simulink model "sim_sim"  (R2018b)
settings: Solver=ode23s  StartTime=0.0  StopTime=T_sweep  RelTol=1e-3
values from neighbouring files (symbols this model uses):
  dgr = 15    [main_sim.m]    (also in main_sim_exp.m = 0.05; main_sim_exp_2.m = 1.5; main_sim_exp_3.m = 0.65; main_sim_exp_4.m = 12)
  dgs = 1    [main_sim.m]    (also in main_sim_exp.m = 3.5; main_sim_exp_2.m = 3.5; main_sim_exp_3.m = 5; main_sim_exp_4.m = 4.25)
  f_log = 1000    [main_sim.m]    (also in main_sim_exp.m; main_sim_exp_2.m; main_sim_exp_3.m; main_sim_exp_4.m)
  I_cur = 2.5    [main_sim.m]
  Jl = 1.2 * Jl    (= 0.0491496)    [main_sim.m]    (also in main_sim_exp.m; main_sim_exp_2.m; main_sim_exp_3.m; main_sim_exp_4.m)
  Jsint = 1.1e-4    (= 0.00011)    [main_sim.m]    (also in main_sim_exp.m; main_sim_exp_2.m; main_sim_exp_3.m; main_sim_exp_4.m)
  Jtot = 1.3*Jtot    (= 0.000159536668197)    [main_sim.m]    (also in main_sim_exp.m = 0.000214342719011; main_sim_exp_2.m = 0.00023185560658; main_sim_exp_3.m = 0.00015903963082; main_sim_exp_4.m = 0.000171808719597)
  kg = 1.15*kg    (= 9660)    [main_sim.m]    (also in main_sim_exp.m; main_sim_exp_2.m = 9240; main_sim_exp_3.m; main_sim_exp_4.m)
  ks = 8.1853e4*1.4    (= 114594.2)    [main_sim.m]    (also in main_sim_exp.m; main_sim_exp_2.m; main_sim_exp_3.m; main_sim_exp_4.m)
  Kt = 53.4e-3    (= 0.0534)    [main_sim.m]    (also in main_sim_exp.m; main_sim_exp_2.m; main_sim_exp_3.m; main_sim_exp_4.m)
  rg = 100    [main_sim.m]    (also in main_sim_exp.m; main_sim_exp_2.m; main_sim_exp_3.m; main_sim_exp_4.m)
  Vel_mot_nom = 391    [main_sim.m]    (also in main_sim_exp.m; main_sim_exp_2.m; main_sim_exp_3.m; main_sim_exp_4.m)
libraries: dspsrcs4 x1, simulink x1
settings Model: Creator=eshojaei  LastModifiedBy=eshojaei
settings CodeAppCC: StateflowObjectComments=on

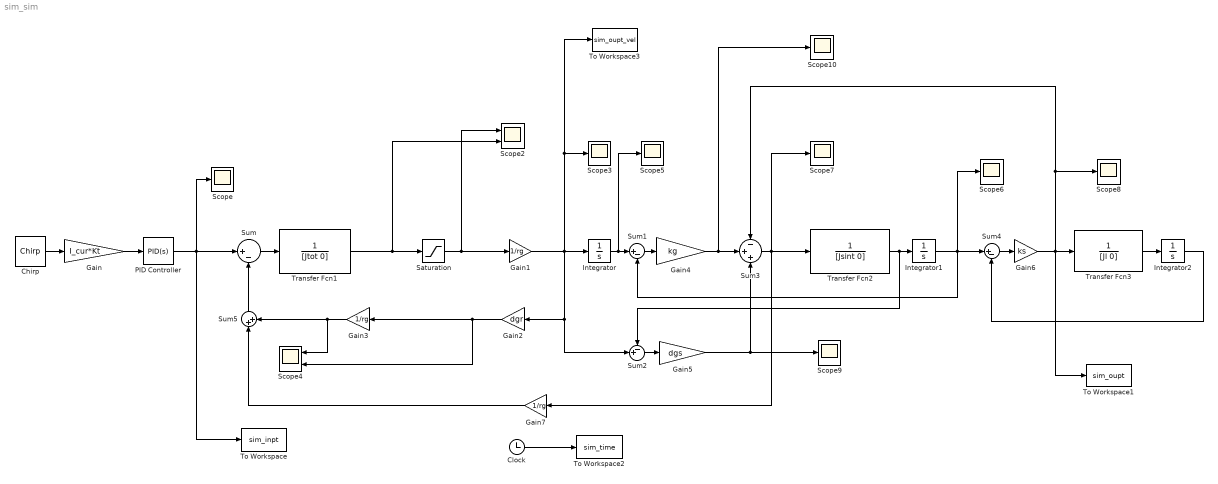
== system sim_sim ==
  Chirp : dspsrcs4/Chirp  sweep=Linear  mode=Unidirectional  f0=f0  f1=f1  t1=T_sweep  Tsweep=T_sweep  phase=0  Ts=1/f_log  spf=1  datatype=Double  OutputFrames=off
      settings: SourceProductName=DSP System Toolbox
  Clock : Clock
  Gain : Gain  Gain=I_cur*Kt
  Gain1 : Gain  Gain=1/rg
  Gain2 : Gain  Gain=dgr
  Gain3 : Gain  Gain=1/rg
  Gain4 : Gain  Gain=kg
  Gain5 : Gain  Gain=dgs
  Gain6 : Gain  Gain=ks
  Gain7 : Gain  Gain=1/rg
  Integrator : Integrator
  Integrator1 : Integrator
  Integrator2 : Integrator
  PID Controller : simulink/Continuous/PID Controller  Controller=PID  Form=Parallel  TimeDomain=Continuous-time  SampleTime=-1  IntegratorMethod=Forward Euler  FilterMethod=Forward Euler  ControllerParametersSource=internal  P=1  I=0  D=0  UseFilter=on  N=100  TunerSelectOption=Transfer Function Based (PID Tuner App)  InitialConditionSource=internal  InitialConditionForIntegrator=0  InitialConditionForFilter=0  DifferentiatorICPrevScaledInput=0  ExternalReset=none  TrackingMode=off  Kt=1  LimitOutput=off  UpperSaturationLimit=inf  LowerSaturationLimit=-inf  LinearizeAsGain=on  AntiWindupMode=none  Kb=1  POutMin=[]  POutMax=[]  IOutMin=[]  IOutMax=[]  DOutMin=[]  DOutMax=[]  NOutMin=[]  NOutMax=[]  SumOutMin=[]  SumOutMax=[]  SaturationOutMin=[]  SaturationOutMax=[]  PParamMin=[]  PParamMax=[]  IParamMin=[]  IParamMax=[]  DParamMin=[]  DParamMax=[]  NParamMin=[]  NParamMax=[]  KbParamMin=[]  KbParamMax=[]  KtParamMin=[]  KtParamMax=[]  KbOutMin=[]  KbOutMax=[]  KtOutMin=[]  KtOutMax=[]  IntegratorOutMin=[]  IntegratorOutMax=[]  FilterOutMin=[]  FilterOutMax=[]  SumI1OutMin=[]  SumI1OutMax=[]  SumI2OutMin=[]  SumI2OutMax=[]  SumI3OutMin=[]  SumI3OutMax=[]  SumI4OutMin=[]  SumI4OutMax=[]  SumDOutMin=[]  SumDOutMax=[]  DifferentiatorOutMin=[]  DifferentiatorOutMax=[]  FilterDiffOutCoefMin=[]  FilterDiffOutCoefMax=[]  ReciprocalOutMin=[]  ReciprocalOutMax=[]  SumDenOutMin=[]  SumDenOutMax=[]  SumNumOutMin=[]  SumNumOutMax=[]  DivideOutMin=[]  DivideOutMax=[]  IntegratorContinuousStateAttributes=''  IntegratorStateMustResolveToSignalObject=off  IntegratorRTWStateStorageClass=Auto  FilterContinuousStateAttributes=''  FilterStateMustResolveToSignalObject=off  FilterRTWStateStorageClass=Auto  ParallelPVariant=InternalParameters  IdealPVariant=Disabled  IVariant=InternalParameters  DVariant=InternalParameters  IntegratorVariant=Continuous  SatVariant=Disabled  AWVariant=Passthrough  PCopyVariant=Disabled  TRVariant=Disabled  FdbkBlocksVariant=Forward  IdealPFdbkVariant=Disabled  SatFdbkVariant=Disabled  DerivativeFilterVariant=ContFilter  NVariant=InternalParameters  NCopyVariant=Disabled  FilterICVariant=InternalICsFilter  IntegratorICVariant=InternalICs  ExternalResetVariant=Disabled  TRSumVariant=Passthrough  SumFdbkVariant=Disabled  SumVariant=Sum_PID
  Saturation : Saturate  UpperLimit=Vel_mot_nom  LowerLimit=-Vel_mot_nom
  Scope{,3,5..10} (8 alike) : Scope
  Scope2 : Scope  NumInputPorts=2
  Scope4 : Scope  NumInputPorts=2
  Sum : Sum  Inputs=|+-
  Sum1 : Sum  Inputs=|+-
  Sum2 : Sum  Inputs=-+|
  Sum3 : Sum  Inputs=-++
  Sum4 : Sum  Inputs=|+-
  Sum5 : Sum  Inputs=|++
  To Workspace : ToWorkspace  VariableName=sim_inpt  SaveFormat=Timeseries  SampleTime=1/f_log
  To Workspace1 : ToWorkspace  VariableName=sim_oupt  SaveFormat=Timeseries  SampleTime=1/f_log
  To Workspace2 : ToWorkspace  VariableName=sim_time  SaveFormat=Timeseries  SampleTime=1/f_log
  To Workspace3 : ToWorkspace  VariableName=sim_oupt_vel  SaveFormat=Timeseries  SampleTime=1/f_log
  Transfer Fcn1 : TransferFcn  Denominator=[Jtot 0]
  Transfer Fcn2 : TransferFcn  Denominator=[Jsint 0]
  Transfer Fcn3 : TransferFcn  Denominator=[Jl 0]
  wires:
  PID Controller/1 -> Sum/1, Scope/1, To Workspace/1
  Transfer Fcn1/1 -> Saturation/1, Scope2/2
  Saturation/1 -> Gain1/1, Scope2/1
  Sum/1 -> Transfer Fcn1/1
  Gain1/1 -> Scope3/1, To Workspace3/1, Integrator/1, Sum2/2, Gain2/1
  Gain2/1 -> Scope4/2, Gain3/1
  Gain3/1 -> Sum5/2, Scope4/1
  Integrator/1 -> Sum1/1, Scope5/1
  Sum1/1 -> Gain4/1
  Transfer Fcn2/1 -> Sum2/1, Integrator1/1
  Integrator1/1 -> Sum4/1, Scope6/1, Sum1/2
  Sum2/1 -> Gain5/1
  Sum3/1 -> Gain7/1, Transfer Fcn2/1, Scope7/1
  Sum4/1 -> Gain6/1
  Transfer Fcn3/1 -> Integrator2/1
  Integrator2/1 -> Sum4/2
  Sum5/1 -> Sum/2
  Clock/1 -> To Workspace2/1
  Gain7/1 -> Sum5/1
  Gain4/1 -> Scope10/1, Sum3/2
  Gain5/1 -> Sum3/3, Scope9/1
  Gain6/1 -> To Workspace1/1, Sum3/1, Scope8/1, Transfer Fcn3/1
  Gain/1 -> PID Controller/1
  Chirp/1 -> Gain/1
